simulink model "prototipo"  (R2022b)
settings: Solver=ode3  StartTime=0.0  StopTime=10  RelTol=1e-3  EnableMultiTasking=on
model workspace (MAT data in the model file):
  RGBData = [62 63 65 64 60 62 65 62 60 59 59 59 ... (230400 elements, 320x240x3)]
libraries: sensehatlib x2, raspberrypiAVlib x2, visionanalysis x1, visiontextngfix x1
(part 1 of 2)
settings Model: FPTRunName=Active  ExtModeTrigDuration=2  Creator=alber  LastModifiedBy=alber
settings SolverCC: AlgebraicLoopSolver=TrustRegion  PositivePriorityOrder=on
settings DataIOCC: LimitDataPoints=on  SaveFormat=Array
settings OptimizationCC: ExpressionDepthLimit=2147483647  ZeroExternalMemoryAtStartup=off  ZeroInternalMemoryAtStartup=off  LifeSpan=Inf  MaxStackSize=64
settings DebuggingCC: UnderspecifiedInitializationDetection=Classic  MergeDetectMultiDrivingBlocksExec=none  FcnCallInpInsideContextMsg=warning  UnconnectedInputMsg=warning  UnconnectedOutputMsg=warning  UnconnectedLineMsg=warning  AllowSymbolicDim=off  StateNameClashWarn=warning  SFUnexpectedBacktrackingDiag=warning  SFNoUnconditionalDefaultTransitionDiag=warning  SFExecutionAtInitializationDiag=none  SFMachineParentedDataDiag=warning  ArithmeticOperatorsInVariantConditions=warning
settings HardwareCC: ProdBitPerPointer=32  ProdBitPerSizeT=32  ProdBitPerPtrDiffT=32  ProdLargestAtomicInteger=Long  ProdLargestAtomicFloat=Double  ProdWordSize=32  ProdHWDeviceType=ARM Compatible->ARM Cortex  UseEmbeddedCoderFeatures=off
settings ModelReferenceCC: EnableRefExpFcnMdlSchedulingChecks=on  PropagateSignalLabelsOutOfModel=off
settings SFSimCC: SimUseLocalCustomCode=off  CustomCodeUndefinedFunction=UseInterfaceOnly
settings RTWCC: Description=Embedded Coder  SystemTargetFile=ert.tlc  HardwareBoard=Raspberry Pi  TemplateMakefile=ert_default_tmf  RTWVerbose=off  RTWUseLocalCustomCode=off  Toolchain=GNU GCC Embedded Linux  BuildConfiguration=Faster Runs  TargetLang=C++  DLTargetLibrary=arm-compute  DLArmComputeVersion=19.05  DLArmComputeArch=armv7
settings CodeAppCC: StateflowObjectComments=on
settings ERTTargetCC: TargetLangStandard=C++03 (ISO)  MultiwordLength=2048  ERTCustomFileBanners=off  CodeInterfacePackaging=C++ class  SupportContinuousTime=on  SupportNonInlinedSFcns=on  RemoveResetFunc=off  SupportVariableSizeSignals=on  ModelStepFunctionPrototypeControlCompliant=off  ConvertIfToSwitch=off  SuppressUnreachableDefaultCases=off
settings ConfigComp: CovMetricSettings=dw  CovSaveCumulativeToWorkspaceVar=on  CovSaveSingleToWorkspaceVar=on  CovExternalEMLEnable=off  CovSFcnEnable=off

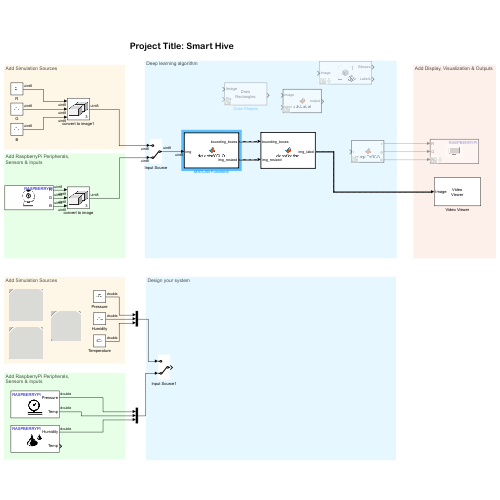
[thumbnail: Simulink's stored preview of the top-level diagram]
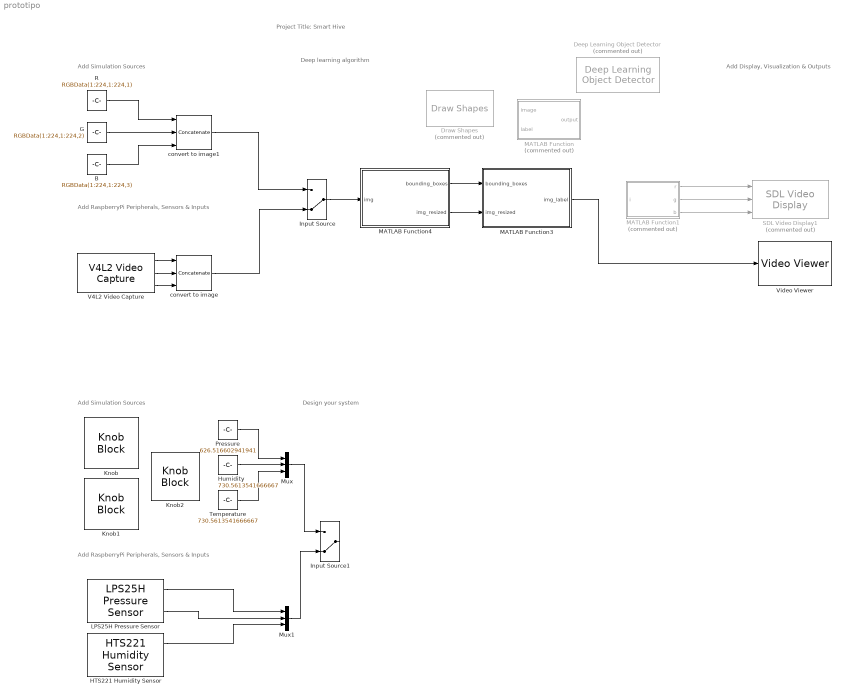
== system prototipo ==
  note: Add Display, Visualization & Outputs
  note: Add Simulation Sources
  note: Project Title: Smart Hive
  note: Deep learning algorithm
  note: Add RaspberryPi Peripherals,
      | Sensors & Inputs
  note: Add Simulation Sources
  note: Add RaspberryPi Peripherals,
      | Sensors & Inputs
  note: Design your system
  B : Constant  Value=RGBData(1:224,1:224,3)  OutDataTypeStr=uint8  SampleTime=0.1
  Deep Learning Object Detector : visionanalysis/Deep Learning Object Detector  Commented=on  Detector=Detector from MAT-file  DetectorFunction=untitled  DetectorFilePath=C:\Users\alber\My Documents\Universidad\4\TFG\Smart Hive\SAVED_OBJECTS\YOLOTY\2\detector.mat  MaxDetections=500  Bboxes=on  Scores=off  UseROI=off  ROI=[1 1 100 100]  Threshold=0.5  NumStrongestRegions=2000  UseMinSize=off  MinSize=[1 1]  UseMaxSize=off  MaxSize=[50 50]  ForceInterpretedSim=off
  Draw Shapes : visiontextngfix/Draw Shapes  Commented=on  shape=Rectangles  fill=off  lineWidth=1  fillClrSource=Specify via dialog  display=Black  intensity=200  color=[200 255 100]  opacity=0.6  viewport=Entire image  antialiasing=off  inType=Obsolete  imagePorts=One multidimensional signal  roundingMode=Floor  overflowMode=off  memoryMode=Specify word length  memoryWordLength=16  prodOutputMode=Binary point scaling  prodOutputWordLength=32  prodOutputFracLength=14  memoryFracLength=15
  G : Constant  Value=RGBData(1:224,1:224,2)  OutDataTypeStr=uint8  SampleTime=0.1
  HTS221 Humidity Sensor : sensehatlib/HTS221 Humidity Sensor  BoardProperty=Pi 2 Model B  OutputDataRate=12.5 Hz  SampleTime=0.1
  Humidity : Constant  Value=730.5613541666667
  Input Source : ManualSwitch  CurrentSetting=0
  Input Source1 : ManualSwitch  CurrentSetting=0
  Knob : KnobBlock  ScaleMax=1024
  Knob1 : KnobBlock  ScaleMax=1024
  Knob2 : KnobBlock  ScaleMax=1024
  LPS25H Pressure Sensor : sensehatlib/LPS25H Pressure Sensor  BoardProperty=Pi 2 Model B  OutputDataRate=25 Hz  SampleTime=0.1
  MATLAB Function : MATLAB Function  Commented=on  TreatAsAtomicUnit=on
  MATLAB Function1 : MATLAB Function  Commented=on  TreatAsAtomicUnit=on
  MATLAB Function3 : MATLAB Function  TreatAsAtomicUnit=on
  MATLAB Function4 : MATLAB Function  TreatAsAtomicUnit=on  VariantControl=Choice
  Mux : Mux  Inputs=3
  Mux1 : Mux  Inputs=3
  Pressure : Constant  Value=626.516602941941
  R : Constant  Value=RGBData(1:224,1:224,1)  OutMin=[224]  OutDataTypeStr=uint8  SampleTime=0.1
  SDL Video Display1 : raspberrypiAVlib/SDL Video Display  Commented=on  title=SDL Video Display  pixelFormat=RGB  pixelOrder=Planar  rowMajor=on  blockPlatform=Raspberry Pi
  Temperature : Constant  Value=730.5613541666667
  V4L2 Video Capture : raspberrypiAVlib/V4L2 Video Capture  DeviceName=/dev/video0  Resolution=custom  CustomResolution=[ 224,224]  PixelFormat=RGB  SampleTime=0.1  pixelOrder=planar  simOutput=Colorbars  imSizeSelection=320x240  imSize=[640, 480]  roi=[0, 0, 640, 480]  m_devName='/dev/video0'  blockPlatform=LINUX  HorizontalFlip=off  VerticalFlip=off  Brightness=0.5  Saturation=0.5  Contrast=0.5  Sharpness=0.5  CameraPan=0  CameraTilt=0  CameraZoom=0.5  EnableManualFocus=on  ManualFocus=0.5
  Video Viewer : VideoViewer  FigPos=[2041 741 418 304]
  convert to image : Concatenate  NumInputs=3  Mode=Multidimensional array  ConcatenateDimension=3
  convert to image1 : Concatenate  NumInputs=3  Mode=Multidimensional array  ConcatenateDimension=3
  wires:
  MATLAB Function1/2(g) -> SDL Video Display1/2
  MATLAB Function1/1(r) -> SDL Video Display1/1
  MATLAB Function1/3(b) -> SDL Video Display1/3
  R/1 -> convert to image1/1
  G/1 -> convert to image1/2
  B/1 -> convert to image1/3
  V4L2 Video Capture/2 -> convert to image/2
  V4L2 Video Capture/1 -> convert to image/1
  V4L2 Video Capture/3 -> convert to image/3
  convert to image1/1 -> Input Source/1
  convert to image/1 -> Input Source/2
  Pressure/1 -> Mux/1
  Humidity/1 -> Mux/2
  Temperature/1 -> Mux/3
  LPS25H Pressure Sensor/1 -> Mux1/1
  HTS221 Humidity Sensor/1 -> Mux1/3
  LPS25H Pressure Sensor/2 -> Mux1/2
  Mux/1 -> Input Source1/1
  Mux1/1 -> Input Source1/2
  MATLAB Function3/1(img_label) -> Video Viewer/1
  Input Source/1 -> MATLAB Function4/1(img)
  MATLAB Function4/1(bounding_boxes) -> MATLAB Function3/1(bounding_boxes)
  MATLAB Function4/2(img_resized) -> MATLAB Function3/2(img_resized)
